simulink model "DialogBoxParameter"  (R2013a)
settings: Solver=ode45  StartTime=0.0  StopTime=10.0  RelTol=1e-3
settings Model: Creator=ajdin  LastModifiedBy=ajdin

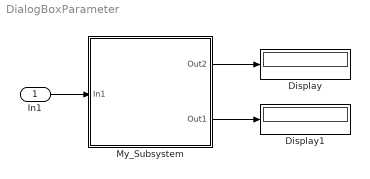
== system DialogBoxParameter ==
  In1 : Inport
  Display : Display
  Display1 : Display
  My_Subsystem : Subsystem  mask{GAIN=87}
      mask init:
      | if(GAIN>5)
      |     Thresh=0.1;
      |     
      | else 
      |     Thresh=0.01;
      |     
      | end
      mask Display:
      | disp('my|sys');
      | color('blue');
      | 
      | port_label('output', 1, 'out');
      | port_label('output', 2, 'Thresh');
      | port_label('input', 1, 'signal');
  wires:
  In1/1 -> My_Subsystem/1(In1)
  My_Subsystem/1(Out2) -> Display/1
  My_Subsystem/2(Out1) -> Display1/1

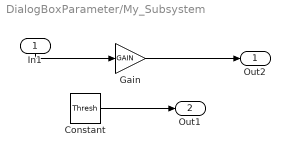
== system DialogBoxParameter/My_Subsystem ==
  In1 : Inport
  Constant : Constant  Value=Thresh
  Gain : Gain  Gain=GAIN
  Out2 : Outport
  Out1 : Outport  Port=2
  wires:
  In1/1 -> Gain/1
  Gain/1 -> Out2/1
  Constant/1 -> Out1/1
